simulink model "System"  (R2020b)
settings: Solver=VariableStepAuto  StartTime=0.0  StopTime=25  RelTol=1e-3
values from neighbouring files (symbols this model uses):
  adapt = 1    [Parameters.m]
  alpha = 1    [Parameters.m]
  c = 100    [Parameters.m]
  k1 = k(1)    [Parameters.m]
  k2 = k(2)    [Parameters.m]
settings Model: Creator=Erfan  LastModifiedBy=Erfan

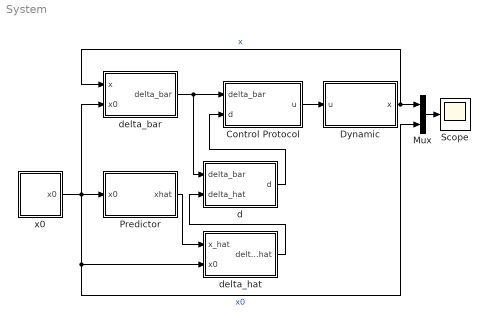
== system System ==
  Control Protocol : Subsystem
  Dynamic : Subsystem
  Mux : Mux  Inputs=2
  Predictor : Subsystem
  Scope : Scope
  d : Subsystem
  delta_bar : Subsystem
  delta_hat : Subsystem
  x0 : Subsystem
  wires:
  x0/1(x0) -> Mux/2, delta_hat/2(x0), delta_bar/2(x0), Predictor/1(x0)  "x0"
  Mux/1 -> Scope/1
  d/1(d) -> Control Protocol/2(d)
  delta_hat/1(delta_hat) -> d/2(delta_hat)
  delta_bar/1(delta_bar) -> d/1(delta_bar), Control Protocol/1(delta_bar)
  Predictor/1(xhat) -> delta_hat/1(x_hat)
  Dynamic/1(x) -> Mux/1, delta_bar/1(x)  "x"
  Control Protocol/1(u) -> Dynamic/1(u)

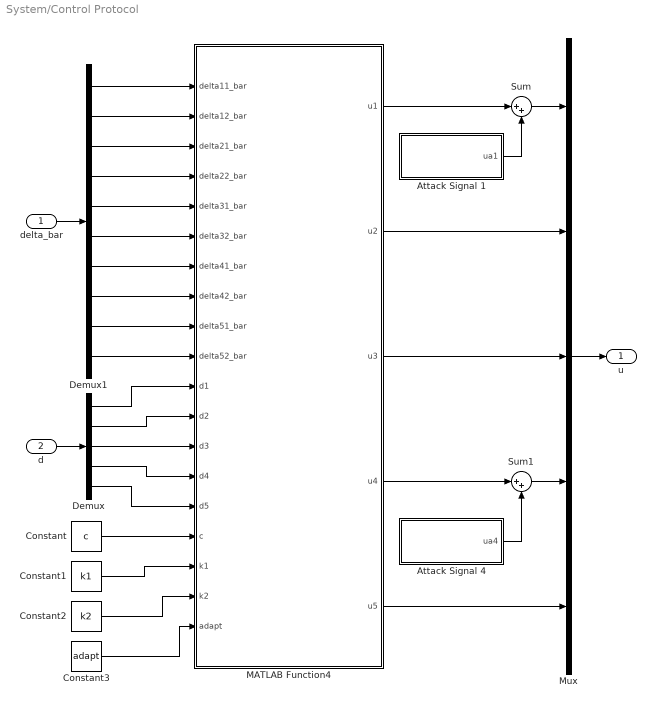
== system System/Control Protocol ==
  delta_bar : Inport
  d : Inport  Port=2
  Attack Signal 1 : Subsystem
  Attack Signal 4 : Subsystem
  Constant : Constant  Value=c
  Constant1 : Constant  Value=k1
  Constant2 : Constant  Value=k2
  Constant3 : Constant  Value=adapt
  Demux : Demux  Outputs=5
  Demux1 : Demux  Outputs=10
  MATLAB Function4 : MATLAB Function  TreatAsAtomicUnit=on
  Mux : Mux  Inputs=5
  Sum : Sum  Inputs=|++
  Sum1 : Sum  Inputs=|++
  u : Outport
  wires:
  MATLAB Function4/3(u3) -> Mux/3
  MATLAB Function4/2(u2) -> Mux/2
  Sum1/1 -> Mux/4
  MATLAB Function4/5(u5) -> Mux/5
  MATLAB Function4/1(u1) -> Sum/1
  MATLAB Function4/4(u4) -> Sum1/1
  Sum/1 -> Mux/1
  Mux/1 -> u/1
  Demux/5 -> MATLAB Function4/15(d5)
  Demux/4 -> MATLAB Function4/14(d4)
  Demux/3 -> MATLAB Function4/13(d3)
  Demux/2 -> MATLAB Function4/12(d2)
  Demux/1 -> MATLAB Function4/11(d1)
  d/1 -> Demux/1
  delta_bar/1 -> Demux1/1
  Demux1/1 -> MATLAB Function4/1(delta11_bar)
  Demux1/2 -> MATLAB Function4/2(delta12_bar)
  Demux1/3 -> MATLAB Function4/3(delta21_bar)
  Demux1/4 -> MATLAB Function4/4(delta22_bar)
  Demux1/5 -> MATLAB Function4/5(delta31_bar)
  Demux1/6 -> MATLAB Function4/6(delta32_bar)
  Demux1/7 -> MATLAB Function4/7(delta41_bar)
  Demux1/8 -> MATLAB Function4/8(delta42_bar)
  Demux1/9 -> MATLAB Function4/9(delta51_bar)
  Demux1/10 -> MATLAB Function4/10(delta52_bar)
  Constant/1 -> MATLAB Function4/16(c)
  Constant1/1 -> MATLAB Function4/17(k1)
  Constant2/1 -> MATLAB Function4/18(k2)
  Attack Signal 1/1(ua1) -> Sum/2
  Attack Signal 4/1(ua4) -> Sum1/2
  Constant3/1 -> MATLAB Function4/19(adapt)

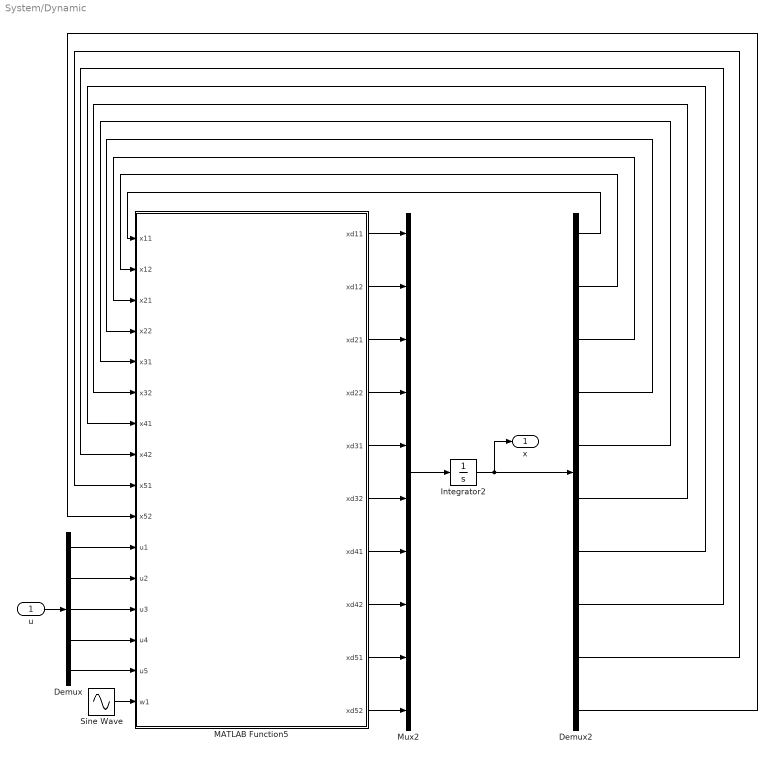
== system System/Dynamic ==
  u : Inport
  Demux : Demux  Outputs=5
  Demux2 : Demux  Outputs=10
  Integrator2 : Integrator  InitialCondition=[1;-1;0;-2;3;2;-3;0;1;-2]
  MATLAB Function5 : MATLAB Function  TreatAsAtomicUnit=on
  Mux2 : Mux  Inputs=10
  Sine Wave : Sin  Amplitude=0.1  Frequency=10  SampleTime=0
  x : Outport
  wires:
  MATLAB Function5/3(xd21) -> Mux2/3
  MATLAB Function5/1(xd11) -> Mux2/1
  MATLAB Function5/5(xd31) -> Mux2/5
  MATLAB Function5/7(xd41) -> Mux2/7
  MATLAB Function5/4(xd22) -> Mux2/4
  MATLAB Function5/10(xd52) -> Mux2/10
  MATLAB Function5/9(xd51) -> Mux2/9
  MATLAB Function5/2(xd12) -> Mux2/2
  MATLAB Function5/8(xd42) -> Mux2/8
  Sine Wave/1 -> MATLAB Function5/16(w1)
  MATLAB Function5/6(xd32) -> Mux2/6
  Integrator2/1 -> Demux2/1, x/1
  Mux2/1 -> Integrator2/1
  Demux/1 -> MATLAB Function5/11(u1)
  Demux/2 -> MATLAB Function5/12(u2)
  Demux/3 -> MATLAB Function5/13(u3)
  Demux/4 -> MATLAB Function5/14(u4)
  Demux/5 -> MATLAB Function5/15(u5)
  u/1 -> Demux/1
  Demux2/1 -> MATLAB Function5/1(x11)
  Demux2/2 -> MATLAB Function5/2(x12)
  Demux2/3 -> MATLAB Function5/3(x21)
  Demux2/4 -> MATLAB Function5/4(x22)
  Demux2/5 -> MATLAB Function5/5(x31)
  Demux2/10 -> MATLAB Function5/10(x52)
  Demux2/9 -> MATLAB Function5/9(x51)
  Demux2/8 -> MATLAB Function5/8(x42)
  Demux2/7 -> MATLAB Function5/7(x41)
  Demux2/6 -> MATLAB Function5/6(x32)

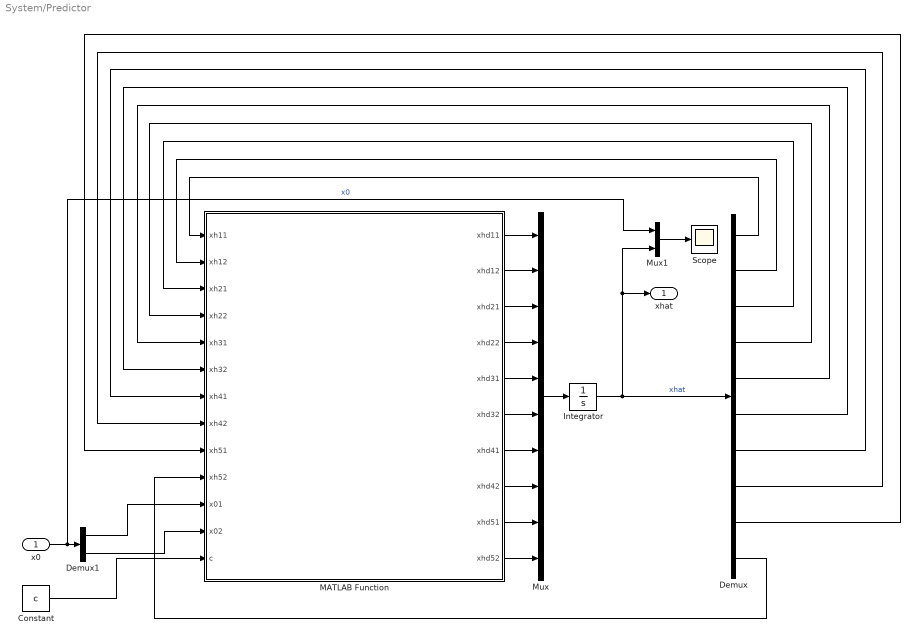
== system System/Predictor ==
  x0 : Inport
  Constant : Constant  Value=c
  Demux : Demux  Outputs=10
  Demux1 : Demux  Outputs=2
  Integrator : Integrator  InitialCondition=[1;-1;0;-2;3;2;-3;0;1;-2]
  MATLAB Function : MATLAB Function  TreatAsAtomicUnit=on
  Mux : Mux  Inputs=10
  Mux1 : Mux  Inputs=2
  Scope : Scope
  xhat : Outport
  wires:
  MATLAB Function/3(xhd21) -> Mux/3
  Integrator/1 -> Demux/1, xhat/1, Mux1/2  "xhat"
  MATLAB Function/2(xhd12) -> Mux/2
  MATLAB Function/7(xhd41) -> Mux/7
  MATLAB Function/5(xhd31) -> Mux/5
  Mux/1 -> Integrator/1
  MATLAB Function/9(xhd51) -> Mux/9
  MATLAB Function/8(xhd42) -> Mux/8
  MATLAB Function/6(xhd32) -> Mux/6
  MATLAB Function/10(xhd52) -> Mux/10
  MATLAB Function/4(xhd22) -> Mux/4
  MATLAB Function/1(xhd11) -> Mux/1
  Demux/1 -> MATLAB Function/1(xh11)
  Demux/2 -> MATLAB Function/2(xh12)
  Demux/3 -> MATLAB Function/3(xh21)
  Demux/4 -> MATLAB Function/4(xh22)
  Demux/10 -> MATLAB Function/10(xh52)
  Demux/9 -> MATLAB Function/9(xh51)
  Demux/8 -> MATLAB Function/8(xh42)
  Demux/7 -> MATLAB Function/7(xh41)
  Demux/6 -> MATLAB Function/6(xh32)
  Demux/5 -> MATLAB Function/5(xh31)
  x0/1 -> Mux1/1, Demux1/1  "x0"
  Demux1/1 -> MATLAB Function/11(x01)
  Demux1/2 -> MATLAB Function/12(x02)
  Mux1/1 -> Scope/1
  Constant/1 -> MATLAB Function/13(c)

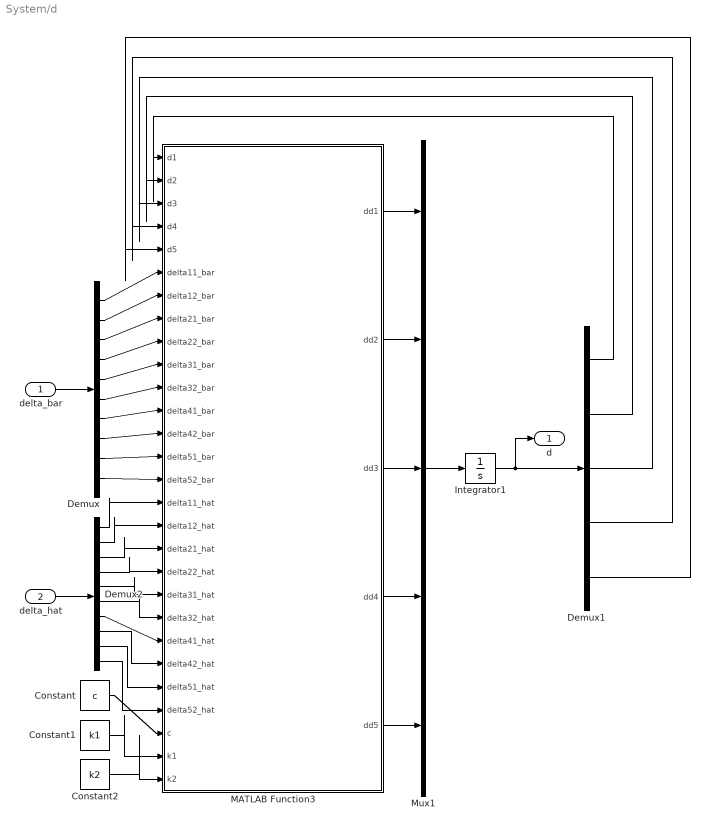
== system System/d ==
  delta_bar : Inport
  delta_hat : Inport  Port=2
  Constant : Constant  Value=c
  Constant1 : Constant  Value=k1
  Constant2 : Constant  Value=k2
  Demux : Demux  Outputs=10
  Demux1 : Demux  Outputs=5
  Demux2 : Demux  Outputs=10
  Integrator1 : Integrator  InitialCondition=[0;0;0;0;0]
  MATLAB Function3 : MATLAB Function  TreatAsAtomicUnit=on
  Mux1 : Mux  Inputs=5
  d : Outport
  wires:
  MATLAB Function3/2(dd2) -> Mux1/2
  MATLAB Function3/4(dd4) -> Mux1/4
  MATLAB Function3/3(dd3) -> Mux1/3
  Integrator1/1 -> Demux1/1, d/1
  MATLAB Function3/5(dd5) -> Mux1/5
  Mux1/1 -> Integrator1/1
  MATLAB Function3/1(dd1) -> Mux1/1
  Demux1/1 -> MATLAB Function3/1(d1)
  Demux1/2 -> MATLAB Function3/2(d2)
  Demux1/3 -> MATLAB Function3/3(d3)
  Demux1/4 -> MATLAB Function3/4(d4)
  Demux1/5 -> MATLAB Function3/5(d5)
  delta_bar/1 -> Demux/1
  Demux/1 -> MATLAB Function3/6(delta11_bar)
  Demux/2 -> MATLAB Function3/7(delta12_bar)
  Demux/3 -> MATLAB Function3/8(delta21_bar)
  Demux/4 -> MATLAB Function3/9(delta22_bar)
  Demux/5 -> MATLAB Function3/10(delta31_bar)
  Demux/6 -> MATLAB Function3/11(delta32_bar)
  Demux/7 -> MATLAB Function3/12(delta41_bar)
  Demux/8 -> MATLAB Function3/13(delta42_bar)
  Demux/9 -> MATLAB Function3/14(delta51_bar)
  Demux/10 -> MATLAB Function3/15(delta52_bar)
  Demux2/10 -> MATLAB Function3/25(delta52_hat)
  Demux2/9 -> MATLAB Function3/24(delta51_hat)
  Demux2/8 -> MATLAB Function3/23(delta42_hat)
  Demux2/7 -> MATLAB Function3/22(delta41_hat)
  Demux2/6 -> MATLAB Function3/21(delta32_hat)
  Demux2/5 -> MATLAB Function3/20(delta31_hat)
  Demux2/4 -> MATLAB Function3/19(delta22_hat)
  Demux2/3 -> MATLAB Function3/18(delta21_hat)
  Demux2/2 -> MATLAB Function3/17(delta12_hat)
  Demux2/1 -> MATLAB Function3/16(delta11_hat)
  delta_hat/1 -> Demux2/1
  Constant/1 -> MATLAB Function3/26(c)
  Constant1/1 -> MATLAB Function3/27(k1)
  Constant2/1 -> MATLAB Function3/28(k2)

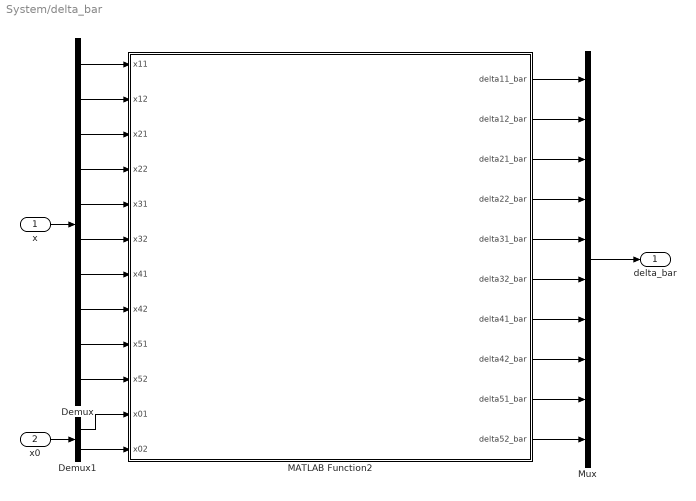
== system System/delta_bar ==
  x : Inport
  x0 : Inport  Port=2
  Demux : Demux  Outputs=10
  Demux1 : Demux  Outputs=2
  MATLAB Function2 : MATLAB Function  TreatAsAtomicUnit=on
  Mux : Mux  Inputs=10
  delta_bar : Outport
  wires:
  x/1 -> Demux/1
  Demux/1 -> MATLAB Function2/1(x11)
  Demux/2 -> MATLAB Function2/2(x12)
  Demux/3 -> MATLAB Function2/3(x21)
  Demux/4 -> MATLAB Function2/4(x22)
  Demux/5 -> MATLAB Function2/5(x31)
  Demux/6 -> MATLAB Function2/6(x32)
  Demux/7 -> MATLAB Function2/7(x41)
  Demux/8 -> MATLAB Function2/8(x42)
  Demux/9 -> MATLAB Function2/9(x51)
  Demux/10 -> MATLAB Function2/10(x52)
  Mux/1 -> delta_bar/1
  MATLAB Function2/1(delta11_bar) -> Mux/1
  MATLAB Function2/2(delta12_bar) -> Mux/2
  MATLAB Function2/3(delta21_bar) -> Mux/3
  MATLAB Function2/4(delta22_bar) -> Mux/4
  MATLAB Function2/5(delta31_bar) -> Mux/5
  MATLAB Function2/6(delta32_bar) -> Mux/6
  MATLAB Function2/7(delta41_bar) -> Mux/7
  MATLAB Function2/8(delta42_bar) -> Mux/8
  MATLAB Function2/9(delta51_bar) -> Mux/9
  MATLAB Function2/10(delta52_bar) -> Mux/10
  Demux1/1 -> MATLAB Function2/11(x01)
  Demux1/2 -> MATLAB Function2/12(x02)
  x0/1 -> Demux1/1

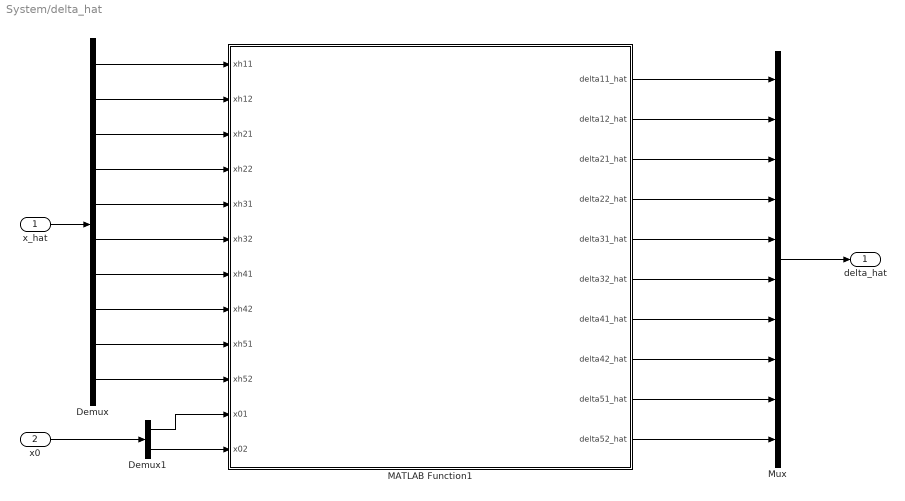
== system System/delta_hat ==
  x_hat : Inport
  x0 : Inport  Port=2
  Demux : Demux  Outputs=10
  Demux1 : Demux  Outputs=2
  MATLAB Function1 : MATLAB Function  TreatAsAtomicUnit=on
  Mux : Mux  Inputs=10
  delta_hat : Outport
  wires:
  Mux/1 -> delta_hat/1
  MATLAB Function1/1(delta11_hat) -> Mux/1
  MATLAB Function1/2(delta12_hat) -> Mux/2
  MATLAB Function1/3(delta21_hat) -> Mux/3
  MATLAB Function1/4(delta22_hat) -> Mux/4
  MATLAB Function1/5(delta31_hat) -> Mux/5
  MATLAB Function1/7(delta41_hat) -> Mux/7
  MATLAB Function1/6(delta32_hat) -> Mux/6
  MATLAB Function1/8(delta42_hat) -> Mux/8
  MATLAB Function1/9(delta51_hat) -> Mux/9
  MATLAB Function1/10(delta52_hat) -> Mux/10
  x_hat/1 -> Demux/1
  Demux/1 -> MATLAB Function1/1(xh11)
  Demux/2 -> MATLAB Function1/2(xh12)
  Demux/3 -> MATLAB Function1/3(xh21)
  Demux/4 -> MATLAB Function1/4(xh22)
  Demux/5 -> MATLAB Function1/5(xh31)
  Demux/6 -> MATLAB Function1/6(xh32)
  Demux/7 -> MATLAB Function1/7(xh41)
  Demux/8 -> MATLAB Function1/8(xh42)
  Demux/9 -> MATLAB Function1/9(xh51)
  Demux/10 -> MATLAB Function1/10(xh52)
  Demux1/1 -> MATLAB Function1/11(x01)
  Demux1/2 -> MATLAB Function1/12(x02)
  x0/1 -> Demux1/1

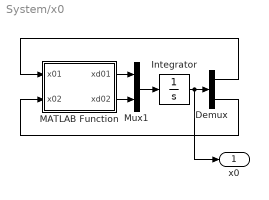
== system System/x0 ==
  Demux : Demux  Outputs=2
  Integrator : Integrator  InitialCondition=[1;-1]
  MATLAB Function : MATLAB Function  TreatAsAtomicUnit=on
  Mux1 : Mux  Inputs=2
  x0 : Outport
  wires:
  MATLAB Function/1(xd01) -> Mux1/1
  Demux/1 -> MATLAB Function/1(x01)
  MATLAB Function/2(xd02) -> Mux1/2
  Integrator/1 -> x0/1, Demux/1
  Mux1/1 -> Integrator/1
  Demux/2 -> MATLAB Function/2(x02)

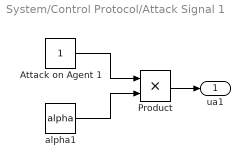
== system System/Control Protocol/Attack Signal 1 ==
  Attack on Agent 1 : Constant
  Product : Product
  alpha1 : Constant  Value=alpha  VectorParams1D=off  SampleTime=-1
  ua1 : Outport
  wires:
  Attack on Agent 1/1 -> Product/1
  alpha1/1 -> Product/2
  Product/1 -> ua1/1

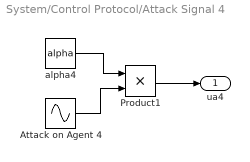
== system System/Control Protocol/Attack Signal 4 ==
  Attack on Agent 4 : Sin  SampleTime=0
  Product1 : Product
  alpha4 : Constant  Value=alpha  VectorParams1D=off  SampleTime=-1
  ua4 : Outport
  wires:
  Product1/1 -> ua4/1
  alpha4/1 -> Product1/1
  Attack on Agent 4/1 -> Product1/2

== matlab function System/d/MATLAB Function3 ==
  data: d1 input; d2 input; d3 input; d4 input; d5 input; delta11_bar input; dd1 output; delta12_bar input; delta21_bar input; delta22_bar input; delta31_bar input; delta32_bar input; delta41_bar input; delta42_bar input; delta51_bar input; delta52_bar input; delta11_hat input; delta12_hat input; delta21_hat input; delta22_hat input; delta31_hat input; delta32_hat input; delta41_hat input; delta42_hat input; delta51_hat input; delta52_hat input; dd2 output; dd3 output; dd4 output; dd5 output; c input; k1 input; k2 input
function [dd1,dd2,dd3,dd4,dd5] = d(d1,d2,d3,d4,d5,delta11_bar,delta12_bar,delta21_bar,delta22_bar,delta31_bar,delta32_bar,delta41_bar,delta42_bar,delta51_bar,delta52_bar,delta11_hat,delta12_hat,delta21_hat,delta22_hat,delta31_hat,delta32_hat,delta41_hat,delta42_hat,delta51_hat,delta52_hat,c,k1,k2)

theta = 20;

dd1 = theta*c*(k1*(delta11_hat - delta11_bar) + k2*(delta12_hat - delta12_bar)) - theta*d1;
dd2 = theta*c*(k1*(delta21_hat - delta21_bar) + k2*(delta22_hat - delta22_bar)) - theta*d2;
dd3 = theta*c*(k1*(delta31_hat - delta31_bar) + k2*(delta32_hat - delta32_bar)) - theta*d3;
dd4 = theta*c*(k1*(delta41_hat - delta41_bar) + k2*(delta42_hat - delta42_bar)) - theta*d4;
dd5 = theta*c*(k1*(delta51_hat - delta51_bar) + k2*(delta52_hat - delta52_bar)) - theta*d5;

== matlab function System/Control Protocol/MATLAB Function4 ==
  data: delta11_bar input; delta12_bar input; delta21_bar input; delta22_bar input; delta31_bar input; delta32_bar input; delta41_bar input; delta42_bar input; delta51_bar input; delta52_bar input; d1 input; u1 output; d2 input; d3 input; d4 input; d5 input; u2 output; u3 output; u4 output; u5 output; c input; k1 input; k2 input; adapt input
function [u1,u2,u3,u4,u5] = Control_Protocol(delta11_bar,delta12_bar,delta21_bar,delta22_bar,delta31_bar,delta32_bar,delta41_bar,delta42_bar,delta51_bar,delta52_bar,d1,d2,d3,d4,d5,c,k1,k2,adapt)

if adapt == 1
    u1 = c*(k1*delta11_bar + k2*delta12_bar) - d1;
    u2 = c*(k1*delta21_bar + k2*delta22_bar) - d2;
    u3 = c*(k1*delta31_bar + k2*delta32_bar) - d3;
    u4 = c*(k1*delta41_bar + k2*delta42_bar) - d4;
    u5 = c*(k1*delta51_bar + k2*delta52_bar) - d5;
else
    u1 = c*(k1*delta11_bar + k2*delta12_bar);
    u2 = c*(k1*delta21_bar + k2*delta22_bar);
    u3 = c*(k1*delta31_bar + k2*delta32_bar);
    u4 = c*(k1*delta41_bar + k2*delta42_bar);
    u5 = c*(k1*delta51_bar + k2*delta52_bar);
end

== matlab function System/Dynamic/MATLAB Function5 ==
  data: x11 input; xd11 output; x12 input; x21 input; x22 input; x31 input; x32 input; x41 input; x42 input; x51 input; x52 input; u1 input; u2 input; u3 input; u4 input; u5 input; w1 input; xd12 output; xd21 output; xd22 output; xd31 output; xd32 output; xd41 output; xd42 output; xd51 output; xd52 output
function [xd11,xd12,xd21,xd22,xd31,xd32,xd41,xd42,xd51,xd52] = Dynamic(x11,x12,x21,x22,x31,x32,x41,x42,x51,x52,u1,u2,u3,u4,u5,w1)

xd11 = x12 + 2*u1 + w1;
xd12 = -x11 + u1 + w1;

xd21 = x22 + 2*u2;
xd22 = -x21 + u2;

xd31 = x32 + 2*u3;
xd32 = -x31 + u3;

xd41 = x42 + 2*u4;
xd42 = -x41 + u4;

xd51 = x52 + 2*u5;
xd52 = -x51 + u5;

== matlab function System/x0/MATLAB Function ==
  data: x01 input; xd01 output; x02 input; xd02 output
function [xd01,xd02] = fcn(x01,x02)

xd01 = x02;
xd02 = -x01;

== matlab function System/delta_hat/MATLAB Function1 ==
  data: xh11 input; delta11_hat output; xh12 input; xh21 input; xh22 input; xh31 input; xh32 input; xh41 input; xh42 input; xh51 input; xh52 input; delta12_hat output; delta21_hat output; delta22_hat output; delta31_hat output; delta32_hat output; delta41_hat output; delta42_hat output; delta51_hat output; delta52_hat output; x01 input; x02 input
function [delta11_hat,delta12_hat,delta21_hat,delta22_hat,delta31_hat,delta32_hat,delta41_hat,delta42_hat,delta51_hat,delta52_hat] = delta_hat(xh11,xh12,xh21,xh22,xh31,xh32,xh41,xh42,xh51,xh52,x01,x02)

delta11_hat = xh31 + xh41 - 2*xh11;
delta12_hat = xh32 + xh42 - 2*xh12;
delta21_hat = xh11 - 2*xh21 + xh31;
delta22_hat = xh12 - 2*xh22 + xh32;
delta31_hat = xh11 - 2*xh31 + x01;
delta32_hat = xh12 - 2*xh32 + x02;
delta41_hat = xh11 - 2*xh41 + xh51;
delta42_hat = xh12 - 2*xh42 + xh52;
delta51_hat = xh21 + xh41 - 2*xh51;
delta52_hat = xh22 + xh42 - 2*xh52;

== matlab function System/Predictor/MATLAB Function ==
  data: xh11 input; xhd11 output; xh12 input; xh21 input; xh22 input; xh31 input; xh32 input; xh41 input; xh42 input; xh51 input; xh52 input; xhd12 output; xhd21 output; xhd22 output; xhd31 output; xhd32 output; xhd41 output; xhd42 output; xhd51 output; xhd52 output; x01 input; x02 input; c input
function [xhd11,xhd12,xhd21,xhd22,xhd31,xhd32,xhd41,xhd42,xhd51,xhd52] = Predictor(xh11,xh12,xh21,xh22,xh31,xh32,xh41,xh42,xh51,xh52,x01,x02,c)

k1 = 1.42;
k2 = -0.02;

xhd11 = xh12 + 2*c*k1*(xh31 + xh41 - 2*xh11) + 2*c*k2*(xh32 + xh42 - 2*xh12);
xhd12 = -xh11 + c*k1*(xh31 + xh41 - 2*xh11) + c*k2*(xh32 + xh42 - 2*xh12);

xhd21 = xh22 + 2*c*k1*(xh11 - 2*xh21 + xh31) + 2*c*k2*(xh12 - 2*xh22 + xh32);
xhd22 = -xh21 + c*k1*(xh11 - 2*xh21 + xh31) + c*k2*(xh12 - 2*xh22 + xh32);

xhd31 = xh32 + 2*c*k1*(xh11 - 2*xh31 + x01) + 2*c*k2*(xh12 - 2*xh32 + x02);
xhd32 = -xh31 + c*k1*(xh11 - 2*xh31 + x01) + c*k2*(xh12 - 2*xh32 + x02);

xhd41 = xh42 + 2*c*k1*(xh11 - 2*xh41 + xh51) + 2*c*k2*(xh12 - 2*xh42 + xh52);
xhd42 = -xh41 + c*k1*(xh11 - 2*xh41 + xh51) + c*k2*(xh12 - 2*xh42 + xh52);

xhd51 = xh52 + 2*c*k1*(xh21 + xh41 - 2*xh51) + 2*c*k2*(xh22 + xh42 - 2*xh52);
xhd52 = -xh51 + c*k1*(xh21 + xh41 - 2*xh51) + c*k2*(xh22 + xh42 - 2*xh52);

== matlab function System/delta_bar/MATLAB Function2 ==
  data: x11 input; delta11_bar output; x12 input; x21 input; x22 input; x31 input; x32 input; x41 input; x42 input; x51 input; x52 input; delta12_bar output; delta21_bar output; delta22_bar output; delta31_bar output; delta32_bar output; delta41_bar output; delta42_bar output; delta51_bar output; delta52_bar output; x01 input; x02 input
function [delta11_bar,delta12_bar,delta21_bar,delta22_bar,delta31_bar,delta32_bar,delta41_bar,delta42_bar,delta51_bar,delta52_bar] = delta_bar(x11,x12,x21,x22,x31,x32,x41,x42,x51,x52,x01,x02)

delta11_bar = x31 + x41 - 2*x11;
delta12_bar = x32 + x42 - 2*x12;
delta21_bar = x11 - 2*x21 + x31;
delta22_bar = x12 - 2*x22 + x32;
delta31_bar = x11 - 2*x31 + x01;
delta32_bar = x12 - 2*x32 + x02;
delta41_bar = x11 - 2*x41 + x51;
delta42_bar = x12 - 2*x42 + x52;
delta51_bar = x21 + x41 - 2*x51;
delta52_bar = x22 + x42 - 2*x52;
